simulink library "ControlAllocationHover"  (R2024a)
settings: Solver=VariableStepAuto  StartTime=0.0  StopTime=10.0  RelTol=1e-3
settings Model: Creator=igmso  LastModifiedBy=igmso

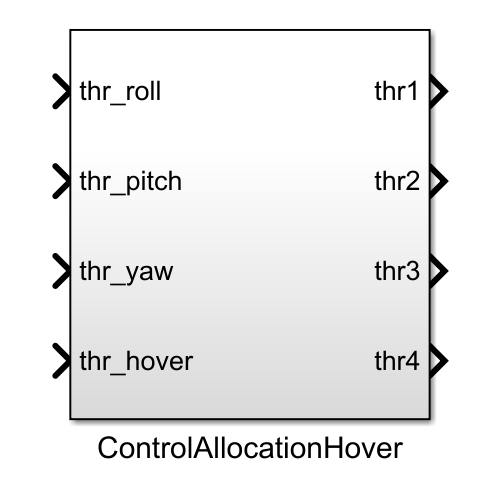
[thumbnail: Simulink's stored preview of the top-level diagram]
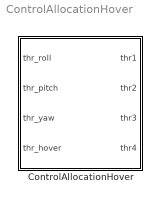
== system ControlAllocationHover ==
  ControlAllocationHover : Subsystem

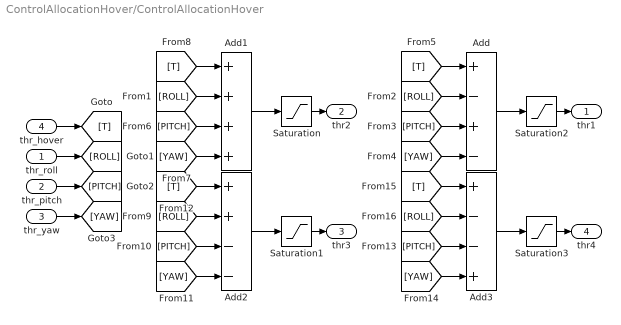
== system ControlAllocationHover/ControlAllocationHover ==
  thr_roll : Inport
  thr_pitch : Inport  Port=2
  thr_yaw : Inport  Port=3
  thr_hover : Inport  Port=4
  Add : Sum  Inputs=+-+-
  Add1 : Sum  Inputs=++++
  Add2 : Sum  Inputs=++--
  Add3 : Sum  Inputs=+--+
  Saturation{,1..3} (4 alike) : Saturate  UpperLimit=1  LowerLimit=0
  thr1 : Outport
  thr2 : Outport  Port=2
  thr3 : Outport  Port=3
  thr4 : Outport  Port=4
  wires:
  Saturation3/1 -> thr4/1
  Saturation2/1 -> thr1/1
  Saturation1/1 -> thr3/1
  Saturation/1 -> thr2/1
  Add3/1 -> Saturation3/1
  Add2/1 -> Saturation1/1
  Add1/1 -> Saturation/1
  Add/1 -> Saturation2/1
  [T] -> Add3/1
  [ROLL] -> Add3/2
  [PITCH] -> Add3/3
  [YAW] -> Add3/4
  [YAW] -> Add2/4
  [PITCH] -> Add2/3
  [ROLL] -> Add2/2
  [T] -> Add2/1
  [T] -> Add1/1
  [ROLL] -> Add1/2
  [PITCH] -> Add1/3
  [YAW] -> Add1/4
  [YAW] -> Add/4
  [PITCH] -> Add/3
  [ROLL] -> Add/2
  [T] -> Add/1
  thr_hover/1 -> [T]
  thr_roll/1 -> [ROLL]
  thr_pitch/1 -> [PITCH]
  thr_yaw/1 -> [YAW]
